simulink model "simulink_discrete_3_R2021a_3"  (R2023b)
settings: Solver=ode45  StartTime=0.0  StopTime=0.7  RelTol=1e-3  EnableMultiTasking=on
undefined symbols (not defined in the file): BW, Ts1, Ts2, Ts3
libraries: cstblocks x12, simulink x5, dspfdesign x2
settings Model: Creator=Koldo  LastModifiedBy=chris
settings SolverCC: AlgebraicLoopSolver=TrustRegion
settings DataIOCC: LimitDataPoints=on  SaveFormat=Array  SignalLoggingSaveFormat=ModelDataLogs  ReturnWorkspaceOutputs=off
settings OptimizationCC: ExpressionDepthLimit=2147483647  LifeSpan=inf
settings DebuggingCC: UnderspecifiedInitializationDetection=Classic  MergeDetectMultiDrivingBlocksExec=none  SolverPrmCheckMsg=warning  FcnCallInpInsideContextMsg=warning  UnconnectedInputMsg=warning  UnconnectedOutputMsg=warning  UnconnectedLineMsg=warning  StateNameClashWarn=warning  SFUnexpectedBacktrackingDiag=warning  SFNoUnconditionalDefaultTransitionDiag=warning  SFExecutionAtInitializationDiag=none  ArithmeticOperatorsInVariantConditions=warning
settings HardwareCC: ProdBitPerPointer=32  ProdBitPerSizeT=32  ProdBitPerPtrDiffT=32  ProdLargestAtomicFloat=None  ProdIntDivRoundTo=Undefined  ProdEndianess=Unspecified  ProdWordSize=32  ProdHWDeviceType=32-bit Generic
settings ModelReferenceCC: EnableRefExpFcnMdlSchedulingChecks=on  PropagateSignalLabelsOutOfModel=off
settings SFSimCC: SimUseLocalCustomCode=off  CustomCodeUndefinedFunction=UseInterfaceOnly
settings RTWCC: RTWUseLocalCustomCode=off  DLArmComputeVersion=19.05
settings CodeAppCC: StateflowObjectComments=on
settings GRTTargetCC: TargetLangStandard=C89/C90 (ANSI)  CombineOutputUpdateFcns=off  GRTInterface=on
settings ConfigComp: CovMetricSettings=dw  CovSaveCumulativeToWorkspaceVar=on  CovSaveSingleToWorkspaceVar=on  CovExternalEMLEnable=off

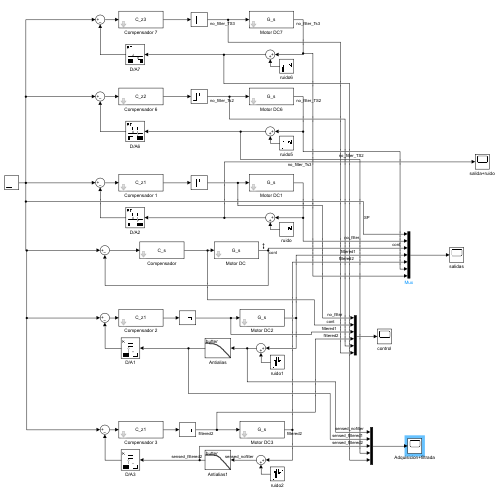
[thumbnail: Simulink's stored preview of the top-level diagram]
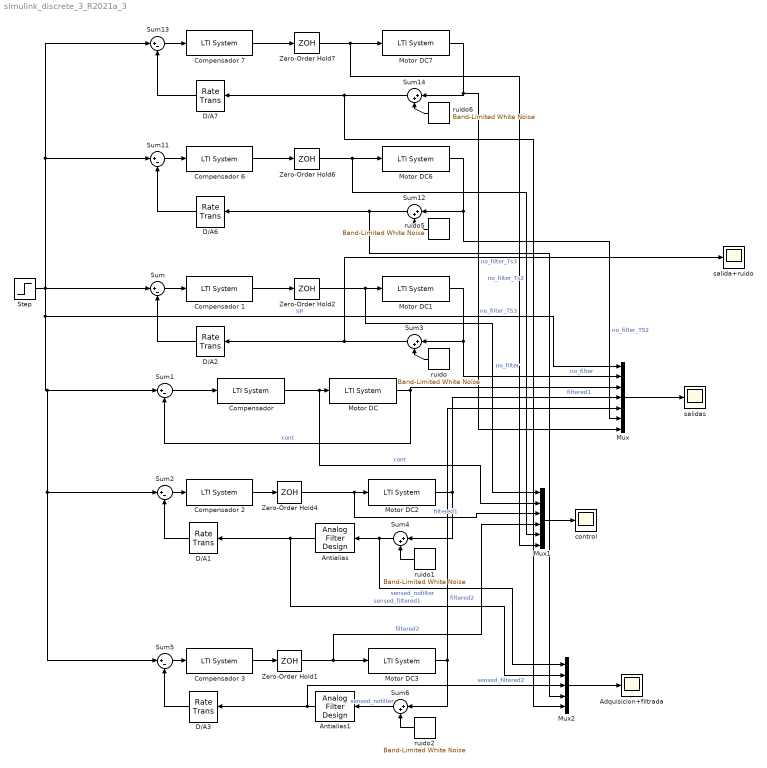
== system simulink_discrete_3_R2021a_3 ==
  Adquisicion+filtrada : Scope
  Antialias : dspfdesign/Analog Filter Design  method=Butterworth  filttype=Lowpass  N=1  Wlo=5*BW  Whi=80  Rp=2  Rs=40
  Antialias1 : dspfdesign/Analog Filter Design  method=Butterworth  filttype=Lowpass  N=2  Wlo=5*BW  Whi=80  Rp=2  Rs=40
  Compensador : cstblocks/LTI System  sys=C_s  IC=[]  PadeOrder=0
  Compensador 1 : cstblocks/LTI System  sys=C_z1  IC=[]  PadeOrder=0
  Compensador 2 : cstblocks/LTI System  sys=C_z1  IC=[]  PadeOrder=0
  Compensador 3 : cstblocks/LTI System  sys=C_z1  IC=[]  PadeOrder=0
  Compensador 6 : cstblocks/LTI System  sys=C_z2  IC=[]  PadeOrder=0
  Compensador 7 : cstblocks/LTI System  sys=C_z3  IC=[]  PadeOrder=0
  D/A1 : RateTransition  Integrity=off  Deterministic=off  InitialCondition=8.96  OutPortSampleTime=Ts1
  D/A2 : RateTransition  Integrity=off  Deterministic=off  InitialCondition=8.96  OutPortSampleTime=Ts1
  D/A3 : RateTransition  Integrity=off  Deterministic=off  InitialCondition=8.96  OutPortSampleTime=Ts1
  D/A6 : RateTransition  Integrity=off  Deterministic=off  InitialCondition=8.96  OutPortSampleTime=Ts2
  D/A7 : RateTransition  Integrity=off  Deterministic=off  InitialCondition=8.96  OutPortSampleTime=Ts3
  "Motor DC " : cstblocks/LTI System  sys=G_s  IC=[]  PadeOrder=0
  Motor DC{1..3,6..7} (5 alike) : cstblocks/LTI System  sys=G_s  IC=[]  PadeOrder=0
  Mux : Mux  Inputs=7
  Mux1 : Mux  Inputs=6
  Mux2 : Mux  Inputs=5
  Step : Step  Time=0.1  After=pi/2  SampleTime=0
  Sum{,1..2,5,11,13} (6 alike) : Sum  Inputs=|+-
  Sum{3..4,6,12,14} (5 alike) : Sum  Inputs=|++
  Zero-Order Hold1 : ZeroOrderHold  SampleTime=Ts1
  Zero-Order Hold2 : ZeroOrderHold  SampleTime=Ts1
  Zero-Order Hold4 : ZeroOrderHold  SampleTime=Ts1
  Zero-Order Hold6 : ZeroOrderHold  SampleTime=Ts2
  Zero-Order Hold7 : ZeroOrderHold  SampleTime=Ts3
  control : Scope
  ruido{,1..2,5..6} (5 alike) : simulink/Sources/Band-Limited White Noise  Cov=[0.0000001]  Ts=0.0001  seed=[23341]
  salida+ruido : Scope
  salidas : Scope
  wires:
  Sum/1 -> Compensador 1/1
  Motor DC1/1 -> Mux/2, Sum3/1  "no_filter"
  Compensador 1/1 -> Zero-Order Hold2/1
  Zero-Order Hold2/1 -> Mux1/1, Motor DC1/1  "no_filter"
  Sum1/1 -> Compensador/1
  "Motor DC "/1 -> Sum1/2, Mux/3  "cont"
  Compensador/1 -> Mux1/2, "Motor DC "/1  "cont"
  Mux/1 -> salidas/1
  Step/1 -> Mux/1, Sum5/1, Sum2/1, Sum1/1, Sum13/1, Sum11/1, Sum/1  "SP"
  Sum2/1 -> Compensador 2/1
  Motor DC2/1 -> Sum4/1, Mux/4  "filtered1"
  Zero-Order Hold4/1 -> Mux1/3, Motor DC2/1  "filtered1"
  Mux1/1 -> control/1
  Compensador 2/1 -> Zero-Order Hold4/1
  Sum3/1 -> salida+ruido/1, D/A2/1
  ruido/1 -> Sum3/2
  Sum4/1 -> Antialias/1, Mux2/1  "sensed_nofilter"
  Antialias/1 -> D/A1/1, Mux2/2  "sensed_filtered1"
  ruido1/1 -> Sum4/2
  Mux2/1 -> Adquisicion+filtrada/1
  D/A2/1 -> Sum/2
  Compensador 3/1 -> Zero-Order Hold1/1
  ruido2/1 -> Sum6/2
  Antialias1/1 -> Mux2/3, D/A3/1  "sensed_filtered2"
  Sum6/1 -> Antialias1/1  "sensed_nofilter"
  D/A3/1 -> Sum5/2
  Zero-Order Hold1/1 -> Mux1/4, Motor DC3/1  "filtered2"
  Motor DC3/1 -> Sum6/1, Mux/5  "filtered2"
  Sum5/1 -> Compensador 3/1
  D/A1/1 -> Sum2/2
  Compensador 6/1 -> Zero-Order Hold6/1
  D/A6/1 -> Sum11/2
  ruido5/1 -> Sum12/2
  Zero-Order Hold6/1 -> Mux1/5, Motor DC6/1  "no_filter_Ts2"
  Sum11/1 -> Compensador 6/1
  Motor DC6/1 -> Mux/6, Sum12/1  "no_filter_TS2"
  Sum12/1 -> Mux2/4, D/A6/1
  Motor DC7/1 -> Mux/7, Sum14/1  "no_filter_Ts3"
  Sum13/1 -> Compensador 7/1
  Zero-Order Hold7/1 -> Mux1/6, Motor DC7/1  "no_filter_TS3"
  ruido6/1 -> Sum14/2
  Sum14/1 -> Mux2/5, D/A7/1
  D/A7/1 -> Sum13/2
  Compensador 7/1 -> Zero-Order Hold7/1
